simulink model "sampleModel1828"  (R2023a)
settings: Solver=VariableStepAuto  StartTime=0.0  StopTime=10.0  RelTol=1e-3
libraries: hdlsllib x5, simulink x2
settings Model: Creator=user1  LastModifiedBy=user1

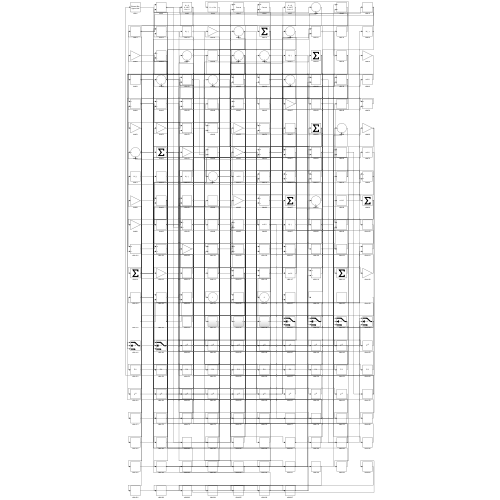
[thumbnail: Simulink's stored preview of the top-level diagram]
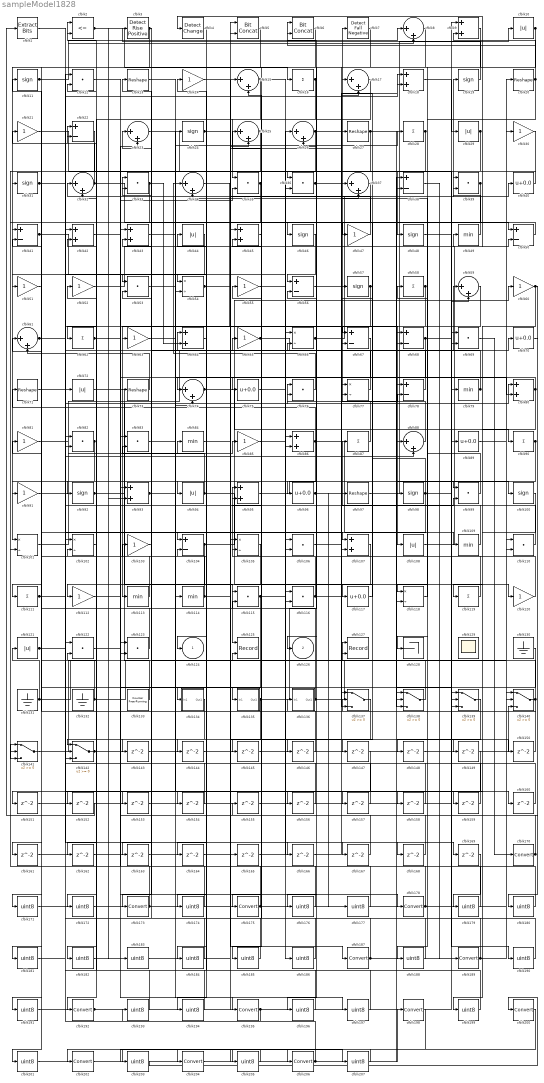
== system sampleModel1828 ==
  cfblk1 : simulink/Logic and Bit Operations/Extract Bits  bitsToExtract=Upper half  numBits=8  bitIdxRange=[0 7]  outScalingMode=Preserve fixed-point scaling
      settings: LibrarySourceBlock=|
      | hdlsllib/Logic and Bit
      | Operations/Extract Bits
  cfblk{10,29,44,72,94,108,121} (7 alike) : Abs  SaturateOnIntegerOverflow=off
  cfblk{11,19,24,31,46,48,57,92,98,100} (10 alike) : Signum
  cfblk{54,66,77,101..102,105,118} (7 alike) : Product  Inputs=*/  RndMeth=Zero  SaturateOnIntegerOverflow=on
  cfblk{14,21,30,47,51..52,55,60,63,65,81,85,91,103,112,120} (16 alike) : Gain
  cfblk{22,38,41,50,56,67..68,78,104} (9 alike) : Sum  Inputs=+-
  cfblk{12,33,35..36,39,53,69,76,82..83,99,106,110,115..116,122..123} (17 alike) : DotProduct  OutDataTypeStr=Inherit: Inherit via internal rule
  cfblk{9,18,42..43,45,64,80,86,93,95,107} (11 alike) : Sum
  cfblk{49,79,84,109,113..114} (6 alike) : MinMax
  cfblk{16,28,58,62,87,90,111,119} (8 alike) : Sum  Inputs=+
  cfblk{40,70,75,89,96,117} (6 alike) : Bias  Bias=0.0  SaturateOnIntegerOverflow=off
  cfblk125 : Record  FileSettingsInternal="{\"entries\":[{\"content\":{\"excelSettings\":{\"content\":{},\"type\":\"Streamout.ExcelSettings\"}},\"type\":\"Streamout.FileSettingStorage\",\"uuid\":\"\"}],\"packageUris\":[\"http:\\/\\/schema.mathworks.com\\/mf0\\/streamout_blocks\\/R2020a\"],\"version\":\"1.0\"}"  Layout=[1 1]  SignalsInternal="{\"entries\":[{\"content\":{\"signals\":[{\"content\":{\"blockPath\":[],\"dimensions\":[1],\"domain\":\"\",\"lineColor\":\"#a2142f\",\"plots\":[1],\"port\":1,\"signalID\":4365,\"signalName\":\"XY Graph:1\"},\"type\":\"RecordBlkView.Signal\",\"uuid\":\"\"},{\"content\":{\"blockPath\":[],\"dimensions\":[1],\"domain\":\"\",\"lineColor\":\"#139fff\",\"plots\":[1],\"port\":2,\"signalID\":4368,\"signalName\":\"XY Graph:2\"},\"type\":\"RecordBlkView.Signal\",\"uuid\":\"\"}]},\"type\":\"RecordBlkView.InputSignals\",\"uuid\":\"\"}],\"packageUris\":[\"http:\\/\\/schema.mathworks.com\\/mf0\\/streamout_blocks\\/R2020a\"],\"version\":\"1.0\"}"  VisualizationBindings="{\"xyplotplugin\":{\"info\":[{\"series\":[{\"bindingParametersList\":[{\"parameter\":\"X-Axis\",\"signalID\":4365,\"signalName\":\"XY Graph:1\"},{\"parameter\":\"Y-Axis\",\"signalID\":4368,\"signalName\":\"XY Graph:2\"}],\"seriesID\":22930}],\"subplotID\":1}]}}"  CompatibilityTag=XY  st=-1
  cfblk127 : Record  FileSettingsInternal="{\"entries\":[{\"content\":{\"excelSettings\":{\"content\":{},\"type\":\"Streamout.ExcelSettings\"}},\"type\":\"Streamout.FileSettingStorage\",\"uuid\":\"\"}],\"packageUris\":[\"http:\\/\\/schema.mathworks.com\\/mf0\\/streamout_blocks\\/R2020a\"],\"version\":\"1.0\"}"  Layout=[1 1]  SignalsInternal="{\"entries\":[{\"content\":{\"signals\":[{\"content\":{\"blockPath\":[],\"dimensions\":[1],\"domain\":\"\",\"lineColor\":\"#a2142f\",\"plots\":[1],\"port\":1,\"signalID\":4373,\"signalName\":\"XY Graph:1\"},\"type\":\"RecordBlkView.Signal\",\"uuid\":\"\"},{\"content\":{\"blockPath\":[],\"dimensions\":[1],\"domain\":\"\",\"lineColor\":\"#139fff\",\"plots\":[1],\"port\":2,\"signalID\":4376,\"signalName\":\"XY Graph:2\"},\"type\":\"RecordBlkView.Signal\",\"uuid\":\"\"}]},\"type\":\"RecordBlkView.InputSignals\",\"uuid\":\"\"}],\"packageUris\":[\"http:\\/\\/schema.mathworks.com\\/mf0\\/streamout_blocks\\/R2020a\"],\"version\":\"1.0\"}"  VisualizationBindings="{\"xyplotplugin\":{\"info\":[{\"series\":[{\"bindingParametersList\":[{\"parameter\":\"X-Axis\",\"signalID\":4373,\"signalName\":\"XY Graph:1\"},{\"parameter\":\"Y-Axis\",\"signalID\":4376,\"signalName\":\"XY Graph:2\"}],\"seriesID\":30710}],\"subplotID\":1}]}}"  CompatibilityTag=XY  st=-1
  cfblk128 : Terminator
  cfblk129 : Scope
      settings: Floating=on
  cfblk{13,20,27,71,73,97} (6 alike) : Reshape
  cfblk130 : Ground
  cfblk131 : Ground
  cfblk132 : Ground
  cfblk133 : hdlsllib/Sources/Counter Free-Running  NumBits=16  tsamp=-1
  cfblk134 : Subsystem
      settings: LibrarySourceBlock=|
      | hdlsllib/Ports &
      | Subsystems/Subsystem
  cfblk135 : Subsystem
      settings: LibrarySourceBlock=|
      | hdlsllib/Ports &
      | Subsystems/Subsystem
  cfblk136 : Subsystem
      settings: LibrarySourceBlock=|
      | hdlsllib/Ports &
      | Subsystems/Subsystem
  cfblk{137..142} (6 alike) : Switch  SaturateOnIntegerOverflow=off  InputSameDT=off
  cfblk{143..169} (27 alike) : Delay  SampleTime=1
  cfblk{8,15,17,23,25..26,32,34,37,59,61,74,88} (13 alike) : Sum  Inputs=|++
  cfblk{170,173,175,178,187,189,192,195,198,200,202,204,206} (13 alike) : DataTypeConversion  SaturateOnIntegerOverflow=off  RndMeth=Floor
  cfblk{171..172,174,176..177,179..186,188,190..191,193..194,196..197,199,201,203,205,207} (25 alike) : DataTypeConversion  OutDataTypeStr=uint8  SaturateOnIntegerOverflow=off  RndMeth=Floor
  cfblk2 : RelationalOperator  Operator=<=  OutDataTypeStr=boolean  InputSameDT=off
  cfblk3 : hdlsllib/Logic and Bit Operations/Detect Rise Positive  vinit=0  OutDataTypeStr=boolean
  cfblk4 : simulink/Logic and Bit Operations/Detect Change  vinit=0  OutDataTypeStr=boolean
      settings: LibrarySourceBlock=|
      | hdlsllib/Logic and Bit
      | Operations/Detect
      | Change
  cfblk5 : hdlsllib/Logic and Bit Operations/Bit Concat  numInputs=2
  cfblk6 : hdlsllib/Logic and Bit Operations/Bit Concat  numInputs=2
  cfblk7 : hdlsllib/Logic and Bit Operations/Detect Fall Negative  vinit=0  OutDataTypeStr=boolean
  cfblk124 : Outport  VectorParamsAs1DForOutWhenUnconnected=off
  cfblk126 : Outport  Port=2  VectorParamsAs1DForOutWhenUnconnected=off
  wires:
  cfblk39/1 -> cfblk126/1, cfblk147/1
  cfblk133/1 -> cfblk76/1
  cfblk135/1(Out1) -> cfblk64/1, cfblk162/1
  cfblk34/1 -> cfblk108/1
  cfblk108/1 -> cfblk4/1
  cfblk100/1 -> cfblk119/1
  cfblk76/1 -> cfblk34/1
  cfblk90/1 -> cfblk158/1, cfblk159/1
  cfblk49/1 -> cfblk19/1
  cfblk50/1 -> cfblk46/1
  cfblk40/1 -> cfblk36/1
  cfblk86/1 -> cfblk109/1, cfblk92/1, cfblk71/1
  cfblk114/1 -> cfblk32/1, cfblk27/1
  cfblk66/1 -> cfblk39/1, cfblk50/2
  cfblk104/1 -> cfblk60/1, cfblk142/1
  cfblk107/1 -> cfblk112/1
  cfblk81/1 -> cfblk15/1
  cfblk17/1 -> cfblk62/1
  cfblk101/1 -> cfblk7/1
  cfblk4/1 -> cfblk134/1(In1)
  cfblk97/1 -> cfblk10/1
  cfblk110/1 -> cfblk87/1
  cfblk43/1 -> cfblk114/1
  cfblk64/1 -> cfblk124/1
  cfblk24/1 -> cfblk54/1, cfblk80/2
  cfblk35/1 -> cfblk94/1, cfblk111/1
  cfblk95/1 -> cfblk100/1
  cfblk52/1 -> cfblk49/1
  cfblk102/1 -> cfblk192/1
  cfblk87/1 -> cfblk37/1
  cfblk54/1 -> cfblk25/2, cfblk144/1
  cfblk16/1 -> cfblk35/1, cfblk172/1
  cfblk140/1 -> cfblk136/1(In1), cfblk33/2, cfblk137/2
  cfblk31/1 -> cfblk53/1, cfblk160/1
  cfblk109/1 -> cfblk17/1
  cfblk119/1 -> cfblk6/1
  cfblk75/1 -> cfblk106/2
  cfblk47/1 -> cfblk2/1
  cfblk59/1 -> cfblk113/1
  cfblk22/1 -> cfblk101/1
  cfblk28/1 -> cfblk101/2, cfblk146/1
  cfblk72/1 -> cfblk125/1
  cfblk98/1 -> cfblk57/1, cfblk150/1, cfblk161/1
  cfblk45/1 -> cfblk175/1
  cfblk80/1 -> cfblk78/1, cfblk199/1
  cfblk92/1 -> cfblk85/1, cfblk35/2
  cfblk141/1 -> cfblk127/1
  cfblk61/1 -> cfblk107/1, cfblk18/2
  cfblk32/1 -> cfblk47/1, cfblk21/1, cfblk137/3
  cfblk25/1 -> cfblk63/1, cfblk82/2, cfblk135/1(In1), cfblk141/3
  cfblk36/1 -> cfblk68/2, cfblk18/1
  cfblk77/1 -> cfblk43/2
  cfblk20/1 -> cfblk9/2, cfblk128/1
  cfblk117/1 -> cfblk77/1
  cfblk136/1(Out1) -> cfblk20/1, cfblk22/2
  cfblk115/1 -> cfblk66/1, cfblk171/1, cfblk174/1
  cfblk116/1 -> cfblk95/1, cfblk78/2
  cfblk33/1 -> cfblk64/2, cfblk141/2, cfblk153/1
  cfblk27/1 -> cfblk138/1, cfblk31/1
  cfblk63/1 -> cfblk28/1
  cfblk23/1 -> cfblk48/1
  cfblk30/1 -> cfblk98/1
  cfblk138/1 -> cfblk125/2
  cfblk111/1 -> cfblk65/1, cfblk66/2, cfblk88/2
  cfblk96/1 -> cfblk99/2, cfblk177/1
  cfblk21/1 -> cfblk139/1
  cfblk113/1 -> cfblk81/1
  cfblk74/1 -> cfblk107/2, cfblk149/1
  cfblk13/1 -> cfblk75/1
  cfblk3/1 -> cfblk41/1, cfblk73/1
  cfblk8/1 -> cfblk96/1
  cfblk94/1 -> cfblk120/1, cfblk33/1, cfblk154/1
  cfblk58/1 -> cfblk74/1, cfblk196/1
  cfblk55/1 -> cfblk26/1
  cfblk68/1 -> cfblk116/2, cfblk59/2
  cfblk123/1 -> cfblk11/1
  cfblk2/1 -> cfblk16/1, cfblk183/1
  cfblk89/1 -> cfblk30/1
  cfblk84/1 -> cfblk39/2
  cfblk18/1 -> cfblk29/1
  cfblk11/1 -> cfblk8/1, cfblk8/2
  cfblk12/1 -> cfblk178/1
  cfblk10/1 -> cfblk77/2, cfblk6/2
  cfblk38/1 -> cfblk189/1
  cfblk131/1 -> cfblk121/1, cfblk86/2
  cfblk1/1 -> cfblk67/1
  cfblk88/1 -> cfblk76/2
  cfblk26/1 -> cfblk51/1, cfblk50/1
  cfblk121/1 -> cfblk80/1, cfblk97/1
  cfblk42/1 -> cfblk195/1
  cfblk78/1 -> cfblk55/1
  cfblk132/1 -> cfblk61/1, cfblk110/2, cfblk22/1
  cfblk60/1 -> cfblk99/1, cfblk180/1
  cfblk112/1 -> cfblk139/2
  cfblk93/1 -> cfblk24/1, cfblk138/3
  cfblk65/1 -> cfblk70/1, cfblk115/1, cfblk90/1
  cfblk106/1 -> cfblk40/1
  cfblk41/1 -> cfblk86/1, cfblk169/1
  cfblk120/1 -> cfblk26/2
  cfblk142/1 -> cfblk74/2, cfblk89/1
  cfblk19/1 -> cfblk3/1
  cfblk14/1 -> cfblk187/1
  cfblk6/1 -> cfblk104/1
  cfblk62/1 -> cfblk93/1, cfblk93/2, cfblk166/1
  cfblk46/1 -> cfblk56/1
  cfblk118/1 -> cfblk58/1
  cfblk103/1 -> cfblk173/1
  cfblk29/1 -> cfblk118/1, cfblk182/1
  cfblk56/1 -> cfblk137/1
  cfblk99/1 -> cfblk34/2
  cfblk69/1 -> cfblk170/1
  cfblk67/1 -> cfblk123/2
  cfblk15/1 -> cfblk139/3, cfblk163/1, cfblk164/1
  cfblk79/1 -> cfblk59/1, cfblk56/2
  cfblk122/1 -> cfblk23/2
  cfblk73/1 -> cfblk61/2
  cfblk91/1 -> cfblk84/1
  cfblk82/1 -> cfblk91/1, cfblk142/3
  cfblk57/1 -> cfblk117/1, cfblk127/2
  cfblk130/1 -> cfblk138/2
  cfblk134/1(Out1) -> cfblk143/1
  cfblk143/1 -> cfblk67/2
  cfblk144/1 -> cfblk68/1
  cfblk7/1 -> cfblk145/1
  cfblk145/1 -> cfblk140/3
  cfblk146/1 -> cfblk41/2
  cfblk139/1 -> cfblk148/1
  cfblk148/1 -> cfblk140/2
  cfblk150/1 -> cfblk25/1
  cfblk51/1 -> cfblk151/1
  cfblk151/1 -> cfblk9/1
  cfblk137/1 -> cfblk152/1
  cfblk152/1 -> cfblk1/1
  cfblk153/1 -> cfblk23/1
  cfblk154/1 -> cfblk142/2
  cfblk70/1 -> cfblk155/1
  cfblk83/1 -> cfblk156/1
  cfblk156/1 -> cfblk116/1
  cfblk53/1 -> cfblk157/1
  cfblk157/1 -> cfblk2/2
  cfblk158/1 -> cfblk106/1
  cfblk159/1 -> cfblk104/2
  cfblk160/1 -> cfblk43/1
  cfblk161/1 -> cfblk54/2
  cfblk162/1 -> cfblk17/2
  cfblk165/1 -> cfblk36/2
  cfblk166/1 -> cfblk37/2
  cfblk85/1 -> cfblk167/1
  cfblk167/1 -> cfblk95/2
  cfblk71/1 -> cfblk168/1
  cfblk168/1 -> cfblk123/1
  cfblk170/1 -> cfblk53/2, cfblk83/2
  cfblk171/1 -> cfblk69/1
  cfblk172/1 -> cfblk69/2
  cfblk173/1 -> cfblk141/1, cfblk83/1
  cfblk174/1 -> cfblk103/1
  cfblk175/1 -> cfblk32/2, cfblk140/1
  cfblk147/1 -> cfblk176/1
  cfblk176/1 -> cfblk45/1
  cfblk177/1 -> cfblk45/2
  cfblk178/1 -> cfblk115/2, cfblk52/1
  cfblk169/1 -> cfblk179/1
  cfblk179/1 -> cfblk12/1
  cfblk180/1 -> cfblk12/2
  cfblk5/1 -> cfblk181/1
  cfblk181/1 -> cfblk72/1
  cfblk182/1 -> cfblk5/1
  cfblk183/1 -> cfblk5/2
  cfblk105/1 -> cfblk184/1
  cfblk184/1 -> cfblk122/1
  cfblk37/1 -> cfblk185/1
  cfblk185/1 -> cfblk105/1
  cfblk155/1 -> cfblk186/1
  cfblk186/1 -> cfblk105/2
  cfblk187/1 -> cfblk122/2, cfblk110/1
  cfblk9/1 -> cfblk188/1
  cfblk188/1 -> cfblk14/1
  cfblk189/1 -> cfblk15/2, cfblk13/1
  cfblk48/1 -> cfblk190/1
  cfblk190/1 -> cfblk38/1
  cfblk149/1 -> cfblk191/1
  cfblk191/1 -> cfblk38/2
  cfblk192/1 -> cfblk165/1, cfblk79/1
  cfblk193/1 -> cfblk102/1
  cfblk164/1 -> cfblk194/1
  cfblk194/1 -> cfblk102/2
  cfblk195/1 -> cfblk193/1, cfblk88/1
  cfblk196/1 -> cfblk42/1
  cfblk163/1 -> cfblk197/1
  cfblk197/1 -> cfblk42/2
  cfblk199/1 -> cfblk44/1
  cfblk44/1 -> cfblk201/1
  cfblk201/1 -> cfblk198/1
  cfblk198/1 -> cfblk203/1
  cfblk203/1 -> cfblk200/1
  cfblk204/1 -> cfblk206/1
  cfblk200/1 -> cfblk205/1
  cfblk205/1 -> cfblk202/1
  cfblk206/1 -> cfblk118/2, cfblk82/1
  cfblk202/1 -> cfblk207/1
  cfblk207/1 -> cfblk204/1

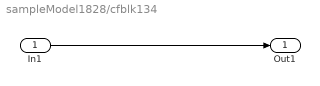
== system sampleModel1828/cfblk134 ==
  In1 : Inport
  Out1 : Outport
  wires:
  In1/1 -> Out1/1

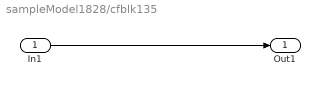
== system sampleModel1828/cfblk135 ==
  In1 : Inport
  Out1 : Outport
  wires:
  In1/1 -> Out1/1

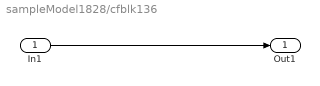
== system sampleModel1828/cfblk136 ==
  In1 : Inport
  Out1 : Outport
  wires:
  In1/1 -> Out1/1
